simulink model "Copy_of_CommonModeSimulation"  (R2023a)
settings: Solver=FixedStepAuto  StartTime=0.0  StopTime=1/ffund  FixedStep=1e-8  RelTol=1e-3
InitFcn:
  | fsw=50e3;
  | 
  | ma=0.8;
  | 
  | ffund=100;
  | 
  | sym= pi/6;
settings Model: Creator=enesa  LastModifiedBy=enesa

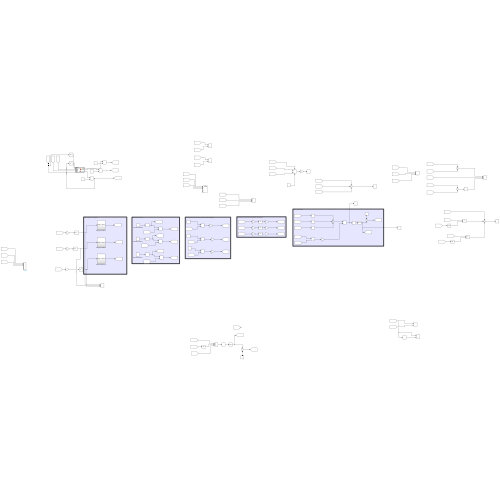
[thumbnail: Simulink's stored preview of the top-level diagram]
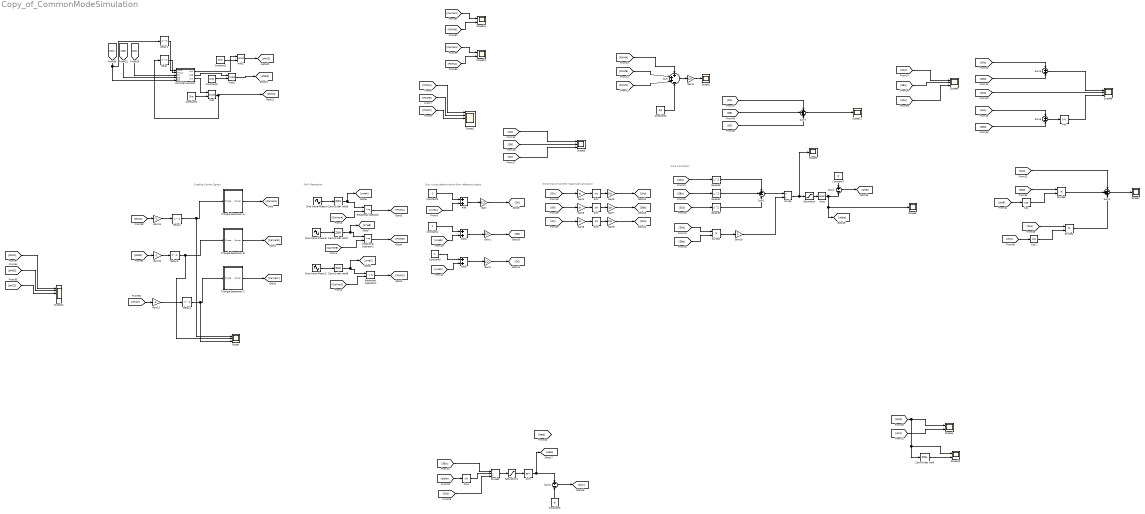
== system Copy_of_CommonModeSimulation ==
  note: Phi B calculation
  note: Switching component magnitude calculation
  note: Duty cycles determination from reference signals
  note: PWM Generation
  note: Creating Carrier Signals
  Abs : Abs  SaturateOnIntegerOverflow=off
  Acos : Trigonometry  Operator=acos
  Add : Sum
  Add1 : Sum
  Add2 : Sum
  Asin : Trigonometry  Operator=asin
  Constant1 : Constant  Value=2*pi
  Constant2 : Constant  Value=2*pi
  Constant3 : Constant
  Constant4 : Constant
  Constant5 : Constant
  Constant6 : Constant  Value=3/2
  Constant7 : Constant  Value=pi
  Constant8 : Constant  Value=pi
  Constant9 : Constant  Value=2*pi
  Cos : Trigonometry  Operator=cos
  Cos1 : Trigonometry  Operator=cos
  Delay{,1..4} (5 alike) : Delay  DelayLength=1  SampleTime=1/fsw
  Divide : Product  Inputs=*/
  Divide1 : Product  Inputs=**
  Divide2 : Product  Inputs=**/
  Divide3 : Product  Inputs=**
  Divide4 : Product  Inputs=**
  Gain : Gain  Gain=1/2
  Gain1 : Gain  Gain=1/2
  Gain10 : Gain  Gain=2
  Gain11 : Gain  Gain=-1
  Gain12 : Gain  Gain=-1
  Gain13 : Gain  Gain=-1
  Gain2 : Gain  Gain=1/2
  Gain3 : Gain  Gain=1/3
  Gain4 : Gain  Gain=pi
  Gain5 : Gain  Gain=2/pi
  Gain6 : Gain  Gain=pi
  Gain7 : Gain  Gain=2/pi
  Gain8 : Gain  Gain=pi
  Gain9 : Gain  Gain=2/pi
  MATLAB Function : MATLAB Function  TreatAsAtomicUnit=on
  Mod : Math  Operator=mod
  Mod1 : Math  Operator=mod
  Mod2 : Math  Operator=mod
  Relational Operator : RelationalOperator  OutDataTypeStr=boolean  RndMeth=Simplest  InputSameDT=off
  Relational Operator1 : RelationalOperator  OutDataTypeStr=boolean  RndMeth=Simplest  InputSameDT=off
  Relational Operator2 : RelationalOperator  OutDataTypeStr=boolean  RndMeth=Simplest  InputSameDT=off
  Saturation : Saturate  UpperLimit=1  LowerLimit=-1
  Saturation1 : Saturate  UpperLimit=1  LowerLimit=-1
  Scope{,3,8..9} (4 alike) : Scope  NumInputPorts=3
  Scope1 : Scope  NumInputPorts=6
  Scope{4,10,13..14} (4 alike) : Scope  NumInputPorts=2
  Scope{2,5..7,11} (5 alike) : Scope
  Scope12 : Scope  NumInputPorts=6
  Sin{1..4} (4 alike) : Trigonometry
  Sine Wave-Phase A : Sin  Amplitude=ma  Frequency=2*pi*ffund  SampleTime=0
  Sine Wave-Phase B : Sin  Amplitude=ma  Frequency=2*pi*ffund  Phase=2*pi/3  SampleTime=0
  Sine Wave-Phase C : Sin  Amplitude=ma  Frequency=2*pi*ffund  Phase=-2*pi/3  SampleTime=0
  Square1 : Math  Operator=square
  Square2 : Math  Operator=square
  Square3 : Math  Operator=square
  Sum : Sum  Inputs=+++-
  Sum1 : Sum  Inputs=++-
  Sum2 : Sum  Inputs=+-
  Sum3 : Sum  Inputs=+-
  Sum4 : Sum  Inputs=+++
  Sum5 : Sum
  Sum6 : Sum  Inputs=+-
  Sum7 : Sum  Inputs=+++
  Triangle Generator-A : Subsystem
  Triangle Generator-B : Subsystem
  Triangle Generator-C : Subsystem
  Zero-Order Hold : ZeroOrderHold  SampleTime=1/fsw
  Zero-Order Hold6 : ZeroOrderHold  SampleTime=5/fsw
  Zero-Order Hold7 : ZeroOrderHold  SampleTime=5/fsw
  Zero-Order Hold8 : ZeroOrderHold  SampleTime=5/fsw
  wires:
  [PWMA] -> Scope1/1
  [PWMB] -> Scope1/2
  [PWMC] -> Scope1/3
  [PWMA] -> Sum/1
  [PWMB] -> Sum/2
  [PWMC] -> Sum/3
  Sum/1 -> Gain3/1
  Gain3/1 -> Scope2/1
  Constant6/1 -> Sum/4
  [DA] -> Scope3/1
  [DB] -> Scope3/2
  [DC] -> Scope3/3
  Triangle Generator-C/1(Carrier) -> [CarrierC]
  Triangle Generator-B/1(Carrier) -> [CarrierB]
  Triangle Generator-A/1(Carrier) -> [CarrierA]
  [CarrierB] -> Relational Operator1/2
  Relational Operator1/1 -> [PWMB]
  Relational Operator/1 -> [PWMA]
  Relational Operator2/1 -> [PWMC]
  [CarrierC] -> Relational Operator2/2
  Sine Wave-Phase A/1 -> Zero-Order Hold6/1
  Sine Wave-Phase C/1 -> Zero-Order Hold8/1
  [CarrierA] -> Relational Operator/2
  Sine Wave-Phase B/1 -> Zero-Order Hold7/1
  [sineC] -> Add2/2
  Constant4/1 -> Add1/1
  Constant3/1 -> Add/1
  Add2/1 -> Gain2/1
  Gain/1 -> [DA]
  Gain2/1 -> [DC]
  Add1/1 -> Gain1/1
  [sineB] -> Add1/2
  Constant5/1 -> Add2/1
  [sineA] -> Add/2
  Gain1/1 -> [DB]
  Add/1 -> Gain/1
  [DA] -> Gain4/1
  Sin1/1 -> Gain5/1
  Gain4/1 -> Sin1/1
  [DB] -> Gain6/1
  Gain7/1 -> [SBp]
  Sin3/1 -> Gain9/1
  Gain6/1 -> Sin2/1
  Gain8/1 -> Sin3/1
  [DC] -> Gain8/1
  Gain5/1 -> [SAp]
  Gain9/1 -> [SCp]
  Sin2/1 -> Gain7/1
  [SCp] -> Square3/1
  Acos/1 -> Sum2/2, Scope6/1, [alpha]
  Gain10/1 -> Divide/2
  Square3/1 -> Sum1/3
  [SAp] -> Divide1/1
  Sum1/1 -> Divide/1
  [SBp] -> Square1/1
  [SBp] -> Divide1/2
  Constant7/1 -> Sum2/1
  Divide/1 -> Scope5/1, Saturation/1
  Square2/1 -> Sum1/1
  [SAp] -> Square2/1
  Sum2/1 -> [phiB]
  Square1/1 -> Sum1/2
  Divide1/1 -> Gain10/1
  [alpha] -> Sin4/1
  [SBp] -> Divide2/1
  Sin4/1 -> Divide2/2
  [SCp] -> Divide2/3
  Divide2/1 -> Saturation1/1
  Asin/1 -> Sum3/1, [beta]
  Constant8/1 -> Sum3/2
  Sum3/1 -> [phic]
  [phiB] -> Scope10/1, Zero-Order Hold/1, Scope4/1
  [phic] -> Scope4/2
  [SBp] -> Divide3/1
  [phiB] -> Cos/1
  Cos/1 -> Divide3/2
  [phic] -> Cos1/1
  Cos1/1 -> Divide4/2
  [SCp] -> Divide4/1
  [SAp] -> Sum4/1
  Divide3/1 -> Sum4/2
  Divide4/1 -> Sum4/3
  Sum4/1 -> Scope7/1
  [SAp] -> Scope8/1
  [SBp] -> Scope8/2
  [SCp] -> Scope8/3
  [SAp] -> Sum5/1
  [SBp] -> Sum5/2
  Sum5/1 -> Scope9/1
  [SCp] -> Scope9/2
  [SAp] -> Sum6/1
  [SBp] -> Sum6/2
  Sum6/1 -> Abs/1
  Abs/1 -> Scope9/3
  Saturation/1 -> Acos/1
  Saturation1/1 -> Asin/1
  Zero-Order Hold/1 -> Scope10/2
  [DA] -> Sum7/1
  [DC] -> Sum7/3
  [DB] -> Sum7/2
  Sum7/1 -> Scope11/1
  [phiB2] -> Scope12/2
  [phiC2] -> Scope12/3
  [DA] -> MATLAB Function/3(DA)
  [DB] -> MATLAB Function/4(DB)
  [DC] -> Delay1/1, MATLAB Function/5(DC)
  [phiA2] -> Scope12/1
  [CarrierA] -> Scope13/1
  [PWMA] -> Scope13/2
  [CarrierA] -> Scope14/1
  [PWMB] -> Scope14/2
  Constant1/1 -> Mod/2
  Constant2/1 -> Mod1/2
  Constant9/1 -> Mod2/2
  Mod2/1 -> [phiB2]
  Mod/1 -> Delay/1, [phiC2]
  Mod1/1 -> [phiA2]
  MATLAB Function/1(phA) -> Mod1/1
  MATLAB Function/2(phB) -> Mod2/1
  MATLAB Function/3(phC) -> Mod/1
  [phiA2] -> Gain11/1
  [phiB2] -> Gain12/1
  [phiC2] -> Gain13/1
  Gain11/1 -> Delay2/1
  Gain13/1 -> Delay4/1
  Zero-Order Hold6/1 -> Relational Operator/1, [sineA]
  Zero-Order Hold7/1 -> [sineB], Relational Operator1/1
  Zero-Order Hold8/1 -> Relational Operator2/1, [sineC]
  Gain12/1 -> Delay3/1
  Delay/1 -> MATLAB Function/2(phC_p)
  Delay1/1 -> MATLAB Function/1(DC_p)
  Delay2/1 -> Scope/1, Triangle Generator-A/1(Phase)
  Delay3/1 -> Scope/2, Triangle Generator-B/1(Phase)
  Delay4/1 -> Scope/3, Triangle Generator-C/1(Phase)

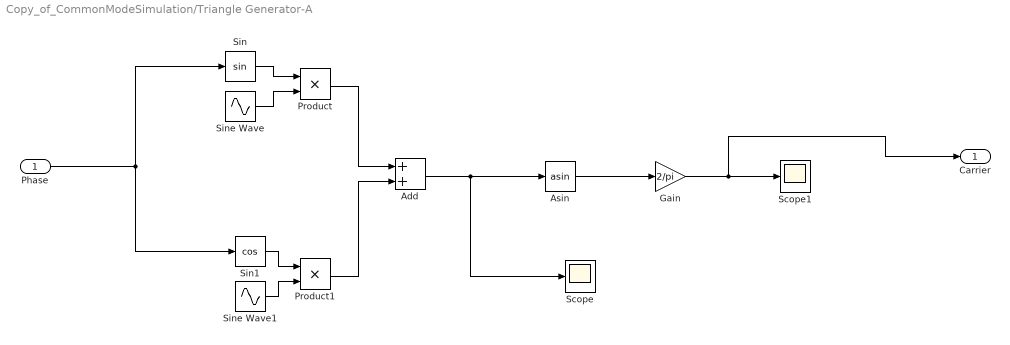
== system Copy_of_CommonModeSimulation/Triangle Generator-A ==
  Phase : Inport
  Add : Sum
  Asin : Trigonometry  Operator=asin
  Gain : Gain  Gain=2/pi
  Product : Product
  Product1 : Product
  Scope : Scope
  Scope1 : Scope
  Sin : Trigonometry
  Sin1 : Trigonometry  Operator=cos
  Sine Wave : Sin  Frequency=2*pi*fsw  SampleTime=0
  Sine Wave1 : Sin  Frequency=2*pi*fsw  Phase=-pi/2  SampleTime=0
  Carrier : Outport
  wires:
  Sin/1 -> Product/1
  Sine Wave/1 -> Product/2
  Phase/1 -> Sin/1, Sin1/1
  Product/1 -> Add/1
  Asin/1 -> Gain/1
  Gain/1 -> Carrier/1, Scope1/1
  Sine Wave1/1 -> Product1/2
  Product1/1 -> Add/2
  Add/1 -> Asin/1, Scope/1
  Sin1/1 -> Product1/1

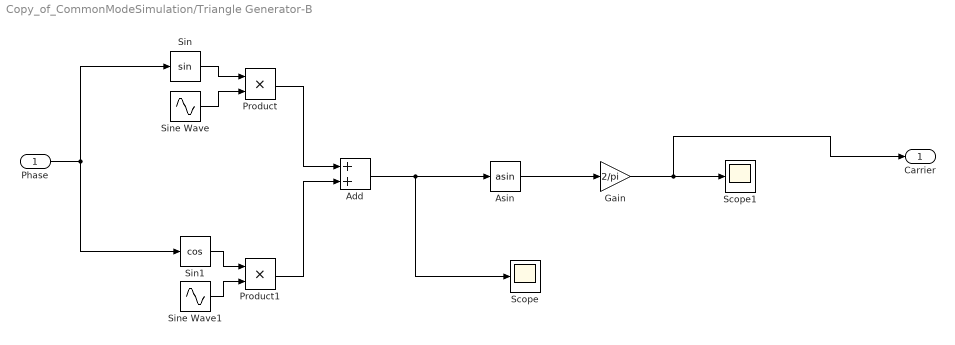
== system Copy_of_CommonModeSimulation/Triangle Generator-B ==
  Phase : Inport
  Add : Sum
  Asin : Trigonometry  Operator=asin
  Gain : Gain  Gain=2/pi
  Product : Product
  Product1 : Product
  Scope : Scope
  Scope1 : Scope
  Sin : Trigonometry
  Sin1 : Trigonometry  Operator=cos
  Sine Wave : Sin  Frequency=2*pi*fsw  SampleTime=0
  Sine Wave1 : Sin  Frequency=2*pi*fsw  Phase=-pi/2  SampleTime=0
  Carrier : Outport
  wires:
  Sin/1 -> Product/1
  Sine Wave/1 -> Product/2
  Phase/1 -> Sin1/1, Sin/1
  Product/1 -> Add/1
  Asin/1 -> Gain/1
  Gain/1 -> Carrier/1, Scope1/1
  Sine Wave1/1 -> Product1/2
  Product1/1 -> Add/2
  Add/1 -> Asin/1, Scope/1
  Sin1/1 -> Product1/1

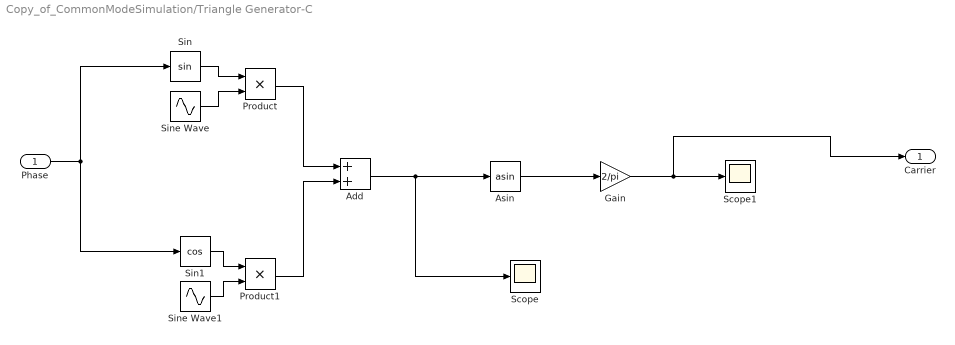
== system Copy_of_CommonModeSimulation/Triangle Generator-C ==
  Phase : Inport
  Add : Sum
  Asin : Trigonometry  Operator=asin
  Gain : Gain  Gain=2/pi
  Product : Product
  Product1 : Product
  Scope : Scope
  Scope1 : Scope
  Sin : Trigonometry
  Sin1 : Trigonometry  Operator=cos
  Sine Wave : Sin  Frequency=2*pi*fsw  SampleTime=0
  Sine Wave1 : Sin  Frequency=2*pi*fsw  Phase=-pi/2  SampleTime=0
  Carrier : Outport
  wires:
  Sin/1 -> Product/1
  Sine Wave/1 -> Product/2
  Phase/1 -> Sin1/1, Sin/1
  Product/1 -> Add/1
  Asin/1 -> Gain/1
  Gain/1 -> Carrier/1, Scope1/1
  Sine Wave1/1 -> Product1/2
  Product1/1 -> Add/2
  Add/1 -> Asin/1, Scope/1
  Sin1/1 -> Product1/1

== matlab function Copy_of_CommonModeSimulation/MATLAB Function ==
  data: DC_p input; phC_p input; DA input; phA output; DB input; DC input; phB output; phC output
function [phA, phB,phC] = fcn(DC_p, phC_p, DA,DB,DC)

phA=phC_p+((DA+DC_p))*pi;
phB=phA+((DA+DB))*pi;
phC= phB+((DB+DC))*pi;

end
